simulink model "MathematicalModel"  (R2018a)
settings: Solver=VariableStepAuto  StartTime=0.0  StopTime=3.0  RelTol=1e-3
values from neighbouring files (symbols this model uses):
  Cds = Coss - Crss    [NumericCalcEx.m]    (also in mathematicalModel.m = 9e-12)
  Cgs = Ciss - Crss    [NumericCalcEx.m]    (also in mathematicalModel.m = 1e-12)
  Lload = 40e-6    (= 4e-05)    [StateSpaceHalfBridge.m]    (also in exStateSpaceHalf.m; mathematicalModel.m = 1e-06)
  Rgg = 3    [mathematicalModel.m]
  Rload = 10    [StateSpaceHalfBridge.m]    (also in exStateSpaceHalf.m; mathematicalModel.m = 100)
  Ron = 6    [mathematicalModel.m]
  Rrc = 10000    [mathematicalModel.m]
  Vdd = 2    [mathematicalModel.m]
  Vgg = 6    [mathematicalModel.m]
  Vth = 1.5    [mathematicalModel.m]
libraries: simulink x1
settings Model: Creator=enes_  LastModifiedBy=enes_

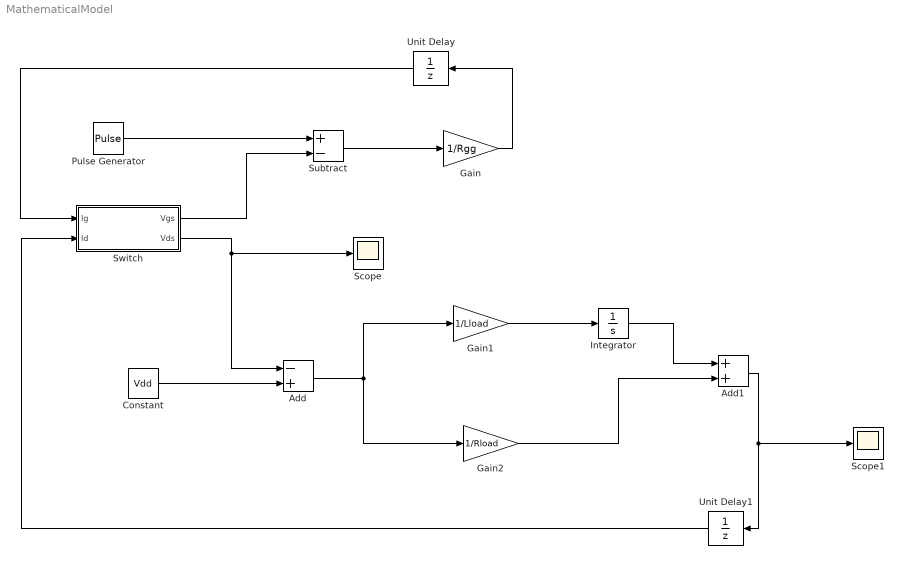
== system MathematicalModel ==
  Add : Sum  Inputs=-+
  Add1 : Sum
  Constant : Constant  Value=Vdd
  Gain : Gain  Gain=1/Rgg
  Gain1 : Gain  Gain=1/Lload
  Gain2 : Gain  Gain=1/Rload
  Integrator : Integrator
  Pulse Generator : DiscretePulseGenerator  PulseType=Time based  Amplitude=Vgg  Period=10e-6  PulseWidth=50
  Scope : Scope
  Scope1 : Scope
  Subtract : Sum  Inputs=+-
  Switch : Subsystem
  Unit Delay : UnitDelay  SampleTime=-1
  Unit Delay1 : UnitDelay  SampleTime=-1
  wires:
  Pulse Generator/1 -> Subtract/1
  Switch/1(Vgs) -> Subtract/2
  Subtract/1 -> Gain/1
  Gain/1 -> Unit Delay/1
  Unit Delay/1 -> Switch/1(Ig)
  Constant/1 -> Add/2
  Add/1 -> Gain2/1, Gain1/1
  Gain1/1 -> Integrator/1
  Integrator/1 -> Add1/1
  Gain2/1 -> Add1/2
  Add1/1 -> Scope1/1, Unit Delay1/1
  Unit Delay1/1 -> Switch/2(Id)
  Switch/2(Vds) -> Scope/1, Add/1

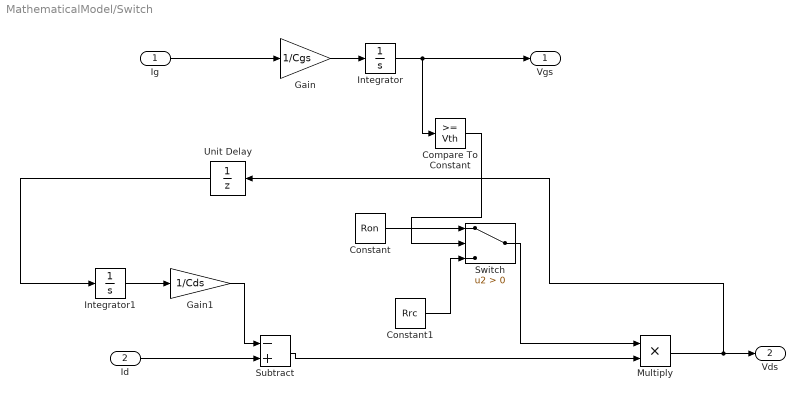
== system MathematicalModel/Switch ==
  Ig : Inport
  Id : Inport  Port=2
  Compare To Constant : simulink/Logic and Bit Operations/Compare To Constant  relop=>=  const=Vth  OutDataTypeStr=boolean
  Constant : Constant  Value=Ron
  Constant1 : Constant  Value=Rrc
  Gain : Gain  Gain=1/Cgs
  Gain1 : Gain  Gain=1/Cds
  Integrator : Integrator
  Integrator1 : Integrator
  Multiply : Product
  Subtract : Sum  Inputs=-+
  Switch : Switch  Criteria=u2 > Threshold
  Unit Delay : UnitDelay  SampleTime=-1
  Vgs : Outport
  Vds : Outport  Port=2
  wires:
  Ig/1 -> Gain/1
  Gain/1 -> Integrator/1
  Integrator/1 -> Compare To Constant/1, Vgs/1
  Id/1 -> Subtract/2
  Integrator1/1 -> Gain1/1
  Gain1/1 -> Subtract/1
  Subtract/1 -> Multiply/2
  Multiply/1 -> Unit Delay/1, Vds/1
  Unit Delay/1 -> Integrator1/1
  Compare To Constant/1 -> Switch/2
  Constant/1 -> Switch/1
  Constant1/1 -> Switch/3
  Switch/1 -> Multiply/1
